simulink model "armSim"  (R2020b)
settings: Solver=ode45  StartTime=0.0  StopTime=5  MaxStep=0.1  MinStep=0.05  RelTol=1e-3
settings Model: Creator=ozelbaz  LastModifiedBy=oze

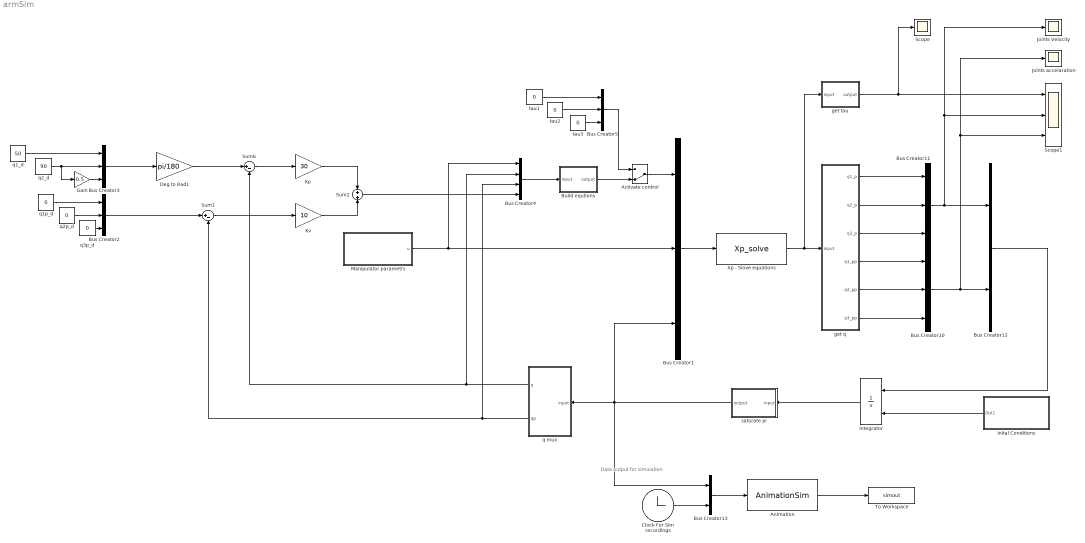
== system armSim ==
  note: Data output for simulation
  Activate control : ManualSwitch  CurrentSetting=0
  Animation : MATLABFcn  Description=yudyu  MATLABFcn=AnimationSim  OutputDimensions=6  OutputSignalType=real
  Build equtions : MATLAB Function  TreatAsAtomicUnit=on
  Bus Creator{1..3,5,10..11} (6 alike) : BusCreator  Inputs=3
  Bus Creator12 : BusCreator  Inputs=2
  Bus Creator13 : BusCreator  Inputs=2
  Bus Creator4 : BusCreator  Inputs=4
  Clock For Sim recordings : Clock
  Deg to Rad1 : Gain  Gain=pi/180
  Gain : Gain  Gain=0.5
  Inital Conditions : Subsystem
  Integrator : Integrator  InitialConditionSource=external
  Joints Velocity : Scope
  Joints accelaration : Scope
  Kp : Gain  Gain=30
  Kv : Gain  Gain=10
  Manipulator parametrs : Subsystem
  Scope : Scope
  Scope1 : Scope  NumInputPorts=3
  Sum1 : Sum  Inputs=|+-
  Sum2 : Sum  Inputs=+|+
  Sum6 : Sum  Inputs=|+-
  To Workspace : ToWorkspace  VariableName=simout  SaveFormat=Timeseries  SampleTime=-1
  Xp - Slove equations : MATLABFcn  Description=yudyu  MATLABFcn=Xp_solve  OutputDimensions=9  OutputSignalType=real
  get q : MATLAB Function  TreatAsAtomicUnit=on
  get tau : MATLAB Function  TreatAsAtomicUnit=on
  q mux : MATLAB Function  TreatAsAtomicUnit=on
  q1_d : Constant  Value=50
  q1p_d : Constant  Value=0
  q2_d : Constant  Value=90
  q2p_d : Constant  Value=0
  q3p_d : Constant  Value=0
  saturate pi : MATLAB Function  TreatAsAtomicUnit=on
  tau1 : Constant  Value=0
  tau2 : Constant  Value=0
  tau3 : Constant  Value=0
  wires:
  tau2/1 -> Bus Creator5/2
  tau1/1 -> Bus Creator5/1
  tau3/1 -> Bus Creator5/3
  get q/1(q1_p) -> Bus Creator11/1
  get q/2(q2_p) -> Bus Creator11/2
  get q/3(q3_p) -> Bus Creator11/3
  get q/4(q1_pp) -> Bus Creator10/1
  get q/5(q2_pp) -> Bus Creator10/2
  get q/6(q3_pp) -> Bus Creator10/3
  Xp - Slove equations/1 -> get tau/1(input), get q/1(input)
  Bus Creator12/1 -> Integrator/1
  Bus Creator1/1 -> Xp - Slove equations/1
  get tau/1(output) -> Scope/1, Scope1/1
  Bus Creator11/1 -> Joints Velocity/1, Scope1/2, Bus Creator12/1
  Bus Creator10/1 -> Joints accelaration/1, Scope1/3, Bus Creator12/2
  Bus Creator13/1 -> Animation/1
  Clock For Sim recordings/1 -> Bus Creator13/2
  Animation/1 -> To Workspace/1
  Manipulator parametrs/1(u) -> Bus Creator1/2, Bus Creator4/1
  Inital Conditions/1(Out1) -> Integrator/2
  Sum1/1 -> Kv/1
  Kp/1 -> Sum2/1
  Bus Creator3/1 -> Deg to Rad1/1
  q3p_d/1 -> Bus Creator2/3
  q2p_d/1 -> Bus Creator2/2
  Bus Creator2/1 -> Sum1/1
  Sum6/1 -> Kp/1
  q1p_d/1 -> Bus Creator2/1
  q2_d/1 -> Gain/1, Bus Creator3/2
  Kv/1 -> Sum2/2
  Gain/1 -> Bus Creator3/3
  Deg to Rad1/1 -> Sum6/1
  q1_d/1 -> Bus Creator3/1
  Integrator/1 -> saturate pi/1(input)
  saturate pi/1(output) -> Bus Creator1/3, q mux/1(input), Bus Creator13/1
  Bus Creator5/1 -> Activate control/1
  Build equtions/1(output) -> Activate control/2
  Activate control/1 -> Bus Creator1/1
  Bus Creator4/1 -> Build equtions/1(input)
  q mux/1(q) -> Bus Creator4/2, Sum6/2
  q mux/2(qp) -> Bus Creator4/3, Sum1/2
  Sum2/1 -> Bus Creator4/4

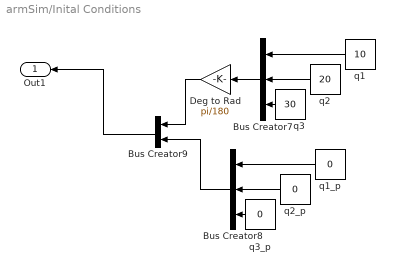
== system armSim/Inital Conditions ==
  Bus Creator7 : BusCreator  Inputs=3
  Bus Creator8 : BusCreator  Inputs=3
  Bus Creator9 : BusCreator  Inputs=2
  Deg to Rad : Gain  Gain=pi/180
  q1 : Constant  Value=10
  q1_p : Constant  Value=0
  q2 : Constant  Value=20
  q2_p : Constant  Value=0
  q3 : Constant  Value=30
  q3_p : Constant  Value=0
  Out1 : Outport
  wires:
  Deg to Rad/1 -> Bus Creator9/1
  Bus Creator7/1 -> Deg to Rad/1
  Bus Creator9/1 -> Out1/1
  q1_p/1 -> Bus Creator8/1
  q2/1 -> Bus Creator7/2
  q2_p/1 -> Bus Creator8/2
  Bus Creator8/1 -> Bus Creator9/2
  q1/1 -> Bus Creator7/1
  q3_p/1 -> Bus Creator8/3
  q3/1 -> Bus Creator7/3

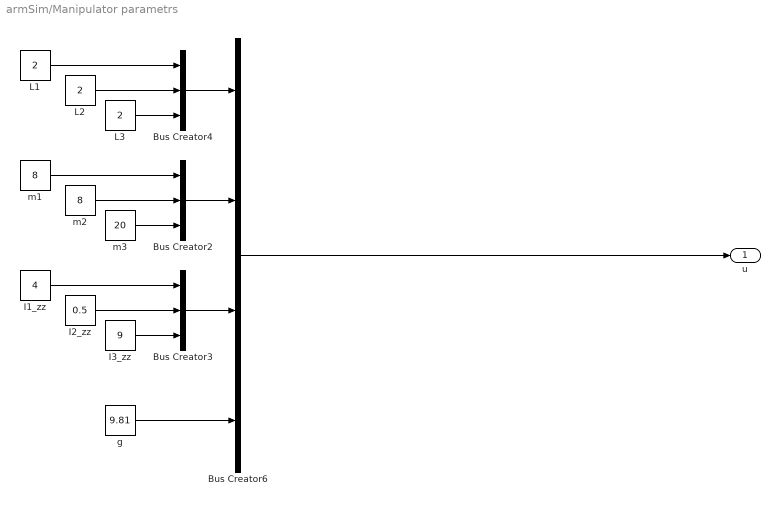
== system armSim/Manipulator parametrs ==
  Bus Creator2 : BusCreator  Inputs=3
  Bus Creator3 : BusCreator  Inputs=3
  Bus Creator4 : BusCreator  Inputs=3
  Bus Creator6 : BusCreator  Inputs=4
  I1_zz : Constant  Value=4
  I2_zz : Constant  Value=0.5
  I3_zz : Constant  Value=9
  L1 : Constant  Value=2
  L2 : Constant  Value=2
  L3 : Constant  Value=2
  g : Constant  Value=9.81
  m1 : Constant  Value=8
  m2 : Constant  Value=8
  m3 : Constant  Value=20
  u : Outport
  wires:
  Bus Creator3/1 -> Bus Creator6/3
  m1/1 -> Bus Creator2/1
  m2/1 -> Bus Creator2/2
  m3/1 -> Bus Creator2/3
  g/1 -> Bus Creator6/4
  I2_zz/1 -> Bus Creator3/2
  Bus Creator6/1 -> u/1
  I1_zz/1 -> Bus Creator3/1
  L1/1 -> Bus Creator4/1
  L2/1 -> Bus Creator4/2
  I3_zz/1 -> Bus Creator3/3
  L3/1 -> Bus Creator4/3
  Bus Creator4/1 -> Bus Creator6/1
  Bus Creator2/1 -> Bus Creator6/2

== matlab function armSim/q mux ==
  data: input input; q output; qp output
function [q, qp]  = q_mux(input)
    q1 = input(1);
    q2 = input(2);
    q3 = input(3);
    q1_p = input(4);
    q2_p = input(5);
    q3_p = input(6);
    q = [q1, q2, q3];
    qp = [q1_p, q2_p, q3_p];
end

== matlab function armSim/get tau ==
  data: input input; output output
function output  = get_tau(input)
    tau1 = input(7);
    tau2 = input(8);
    tau3 = input(9);
    output = [tau1, tau2, tau3];
end

== matlab function armSim/saturate pi ==
  data: input input; output output
function output  = saturate_pi(input)
    q1 = input(1);
    q2 = input(2);
    q3 = input(3);
    q1_p = input(4);
    q2_p = input(5);
    q3_p = input(6); 
    q1 = atan2(sin(q1),cos(q1));
    q2 = atan2(sin(q2),cos(q2));
    q3 = atan2(sin(q3),cos(q3));
    output = [q1, q2, q3, q1_p, q2_p, q3_p];
end

== matlab function armSim/get q ==
  data: input input; q1_p output; q2_p output; q3_p output; q1_pp output; q2_pp output; q3_pp output
function [q1_p, q2_p, q3_p, q1_pp, q2_pp, q3_pp]  = get_q(input)
    q1_p = input(1);
    q2_p = input(2);
    q3_p = input(3);
    q1_pp = input(4);
    q2_pp = input(5);
    q3_pp = input(6);
    %output = [q1_p, q2_p, q3_p, q1_pp, q2_pp, q3_pp];
end

== matlab function armSim/Build equtions ==
  data: input input; output output
function output = fcn(input)

    L1 = input(1);
    L2 = input(2);
    L3 = input(3);
    m1 = input(4);
    m2 = input(5);
    m3 = input(6);
    I1_zz = input(7);
    I2_zz = input(8);
    I3_zz = input(9);
    g = input(10);
    %D1 = input(11);
    %D2 = input(12);
    %D3 = input(13);
%     D1 = 1;
%     D2 = 1;
%     D3 = 1;
    q1 = input(11);
    q2 = input(12);
    q3 = input(13);
    q1_p = input(14);
    q2_p = input(15);
    q3_p = input(16);
    q1_pp = input(17);
    q2_pp = input(18);
    q3_pp = input(19);

%     tau1_act = D1*q1_p + q3_pp*(I3_zz + (L3^2*m3)/4 + (L1*L3*m3*cos(q2 + q3))/2 + (L2*L3*m3*cos(q3))/2) + q1_pp*(I1_zz + I2_zz + I3_zz + (L1^2*m1)/4 + L1^2*m2 + L1^2*m3 + (L2^2*m2)/4 + L2^2*m3 + (L3^2*m3)/4 + L1*L3*m3*cos(q2 + q3) + L1*L2*m2*cos(q2) + 2*L1*L2*m3*cos(q2) + L2*L3*m3*cos(q3)) + (5*g*(7*L2*cos(q1 + q2) + 14*L1*cos(q1) + 2*L3*cos(q1 + q2 + q3)))/2 + q2_pp*(I2_zz + I3_zz + (L2^2*m2)/4 + L2^2*m3 + (L3^2*m3)/4 + (L1*L3*m3*cos(q2 + q3))/2 + (L1*L2*m2*cos(q2))/2 + L1*L2*m3*cos(q2) + L2*L3*m3*cos(q3)) - (L1*q2_p^2*(L3*m3*sin(q2 + q3) + L2*m2*sin(q2) + 2*L2*m3*sin(q2)))/2 - (L3*m3*q3_p^2*(L1*sin(q2 + q3) + L2*sin(q3)))/2 - L1*q1_p*q2_p*(L3*m3*sin(q2 + q3) + L2*m2*sin(q2) + 2*L2*m3*sin(q2)) - L3*m3*q1_p*q3_p*(L1*sin(q2 + q3) + L2*sin(q3)) - L3*m3*q2_p*q3_p*(L1*sin(q2 + q3) + L2*sin(q3));
%     tau2_act = D2*q2_p + I2_zz*q1_pp + I2_zz*q2_pp + I3_zz*q1_pp + I3_zz*q2_pp + I3_zz*q3_pp + 5*L3*g*cos(q1 + q2 + q3) + (35*L2*g*cos(q1 + q2))/2 + (L2^2*m2*q1_pp)/4 + (L2^2*m2*q2_pp)/4 + L2^2*m3*q1_pp + L2^2*m3*q2_pp + (L3^2*m3*q1_pp)/4 + (L3^2*m3*q2_pp)/4 + (L3^2*m3*q3_pp)/4 + (L1*L2*m2*q1_p^2*sin(q2))/2 + L1*L2*m3*q1_p^2*sin(q2) - (L2*L3*m3*q3_p^2*sin(q3))/2 + (L1*L3*m3*q1_pp*cos(q2 + q3))/2 + (L1*L2*m2*q1_pp*cos(q2))/2 + L1*L2*m3*q1_pp*cos(q2) + L2*L3*m3*q1_pp*cos(q3) + L2*L3*m3*q2_pp*cos(q3) + (L2*L3*m3*q3_pp*cos(q3))/2 + (L1*L3*m3*q1_p^2*sin(q2 + q3))/2 - L2*L3*m3*q1_p*q3_p*sin(q3) - L2*L3*m3*q2_p*q3_p*sin(q3);
%     tau3_act = (L3*m3*(L1*sin(q2 + q3) + L2*sin(q3))*q1_p^2)/2 + L2*L3*m3*sin(q3)*q1_p*q2_p + (L2*L3*m3*sin(q3)*q2_p^2)/2 + D3*q3_p + q2_pp*((m3*L3^2)/4 + (L2*m3*cos(q3)*L3)/2 + I3_zz) + q1_pp*(I3_zz + (L3^2*m3)/4 + (L1*L3*m3*cos(q2 + q3))/2 + (L2*L3*m3*cos(q3))/2) + q3_pp*((m3*L3^2)/4 + I3_zz) + 5*L3*g*cos(q1 + q2 + q3);

    tau1_act = I1_zz*q1_pp + I2_zz*q1_pp + I2_zz*q2_pp + I3_zz*q1_pp + I3_zz*q2_pp + I3_zz*q3_pp + (6867*L2*cos(q1 + q2))/40 + (6867*L1*cos(q1))/20 + (981*L3*cos(q1 + q2 + q3))/20 + (L1^2*m1*q1_pp)/4 + L1^2*m2*q1_pp + L1^2*m3*q1_pp + (L2^2*m2*q1_pp)/4 + (L2^2*m2*q2_pp)/4 + L2^2*m3*q1_pp + L2^2*m3*q2_pp + (L3^2*m3*q1_pp)/4 + (L3^2*m3*q2_pp)/4 + (L3^2*m3*q3_pp)/4 - (L1*L2*m2*q2_p^2*sin(q2))/2 - L1*L2*m3*q2_p^2*sin(q2) - (L2*L3*m3*q3_p^2*sin(q3))/2 + L1*L3*m3*q1_pp*cos(q2 + q3) + (L1*L3*m3*q2_pp*cos(q2 + q3))/2 + (L1*L3*m3*q3_pp*cos(q2 + q3))/2 + L1*L2*m2*q1_pp*cos(q2) + (L1*L2*m2*q2_pp*cos(q2))/2 + 2*L1*L2*m3*q1_pp*cos(q2) + L1*L2*m3*q2_pp*cos(q2) + L2*L3*m3*q1_pp*cos(q3) + L2*L3*m3*q2_pp*cos(q3) + (L2*L3*m3*q3_pp*cos(q3))/2 - (L1*L3*m3*q2_p^2*sin(q2 + q3))/2 - (L1*L3*m3*q3_p^2*sin(q2 + q3))/2 - L1*L2*m2*q1_p*q2_p*sin(q2) - 2*L1*L2*m3*q1_p*q2_p*sin(q2) - L2*L3*m3*q1_p*q3_p*sin(q3) - L2*L3*m3*q2_p*q3_p*sin(q3) - L1*L3*m3*q1_p*q2_p*sin(q2 + q3) - L1*L3*m3*q1_p*q3_p*sin(q2 + q3) - L1*L3*m3*q2_p*q3_p*sin(q2 + q3);
    tau2_act = I2_zz*q1_pp + I2_zz*q2_pp + I3_zz*q1_pp + I3_zz*q2_pp + I3_zz*q3_pp + (6867*L2*cos(q1 + q2))/40 + (981*L3*cos(q1 + q2 + q3))/20 + (L2^2*m2*q1_pp)/4 + (L2^2*m2*q2_pp)/4 + L2^2*m3*q1_pp + L2^2*m3*q2_pp + (L3^2*m3*q1_pp)/4 + (L3^2*m3*q2_pp)/4 + (L3^2*m3*q3_pp)/4 + (L1*L2*m2*q1_p^2*sin(q2))/2 + L1*L2*m3*q1_p^2*sin(q2) - (L2*L3*m3*q3_p^2*sin(q3))/2 + (L1*L3*m3*q1_pp*cos(q2 + q3))/2 + (L1*L2*m2*q1_pp*cos(q2))/2 + L1*L2*m3*q1_pp*cos(q2) + L2*L3*m3*q1_pp*cos(q3) + L2*L3*m3*q2_pp*cos(q3) + (L2*L3*m3*q3_pp*cos(q3))/2 + (L1*L3*m3*q1_p^2*sin(q2 + q3))/2 - L2*L3*m3*q1_p*q3_p*sin(q3) - L2*L3*m3*q2_p*q3_p*sin(q3);
    tau3_act = I3_zz*q1_pp + I3_zz*q2_pp + I3_zz*q3_pp + (981*L3*cos(q1 + q2 + q3))/20 + (L3^2*m3*q1_pp)/4 + (L3^2*m3*q2_pp)/4 + (L3^2*m3*q3_pp)/4 + (L2*L3*m3*q1_p^2*sin(q3))/2 + (L2*L3*m3*q2_p^2*sin(q3))/2 + (L1*L3*m3*q1_pp*cos(q2 + q3))/2 + (L2*L3*m3*q1_pp*cos(q3))/2 + (L2*L3*m3*q2_pp*cos(q3))/2 + (L1*L3*m3*q1_p^2*sin(q2 + q3))/2 + L2*L3*m3*q1_p*q2_p*sin(q3);
    
    output = [tau1_act, tau2_act, tau3_act];
end
